simulink model "sysID_1"  (R2024a)
settings: Solver=VariableStepAuto  StartTime=0.0  StopTime=T + Ttrans  RelTol=1e-3
undefined symbols (not defined in the file): K, N, omega0, T, Ts
settings Model: Creator=dunni  LastModifiedBy=dunni

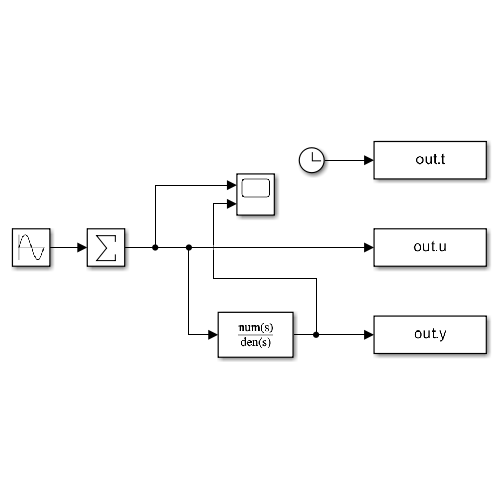
[thumbnail: Simulink's stored preview of the top-level diagram]
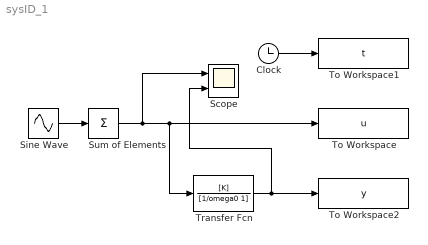
== system sysID_1 ==
  Clock : Clock
  Scope : Scope  NumInputPorts=2
  Sine Wave : Sin  Frequency=(1:N)*2*pi/T  Phase=2*pi.*rand(1,N)  SampleTime=0
  Sum of Elements : Sum  Inputs=+
  To Workspace : ToWorkspace  VariableName=u  SampleTime=Ts
      settings: MaxDataPoints=T/Ts
  To Workspace1 : ToWorkspace  VariableName=t  SampleTime=Ts
      settings: MaxDataPoints=T/Ts
  To Workspace2 : ToWorkspace  VariableName=y  SampleTime=Ts
      settings: MaxDataPoints=T/Ts
  Transfer Fcn : TransferFcn  Numerator=[K]  Denominator=[1/omega0 1]
  wires:
  Sine Wave/1 -> Sum of Elements/1
  Clock/1 -> To Workspace1/1
  Transfer Fcn/1 -> Scope/2, To Workspace2/1
  Sum of Elements/1 -> Transfer Fcn/1, To Workspace/1, Scope/1
